simulink model "quadcopter_control_2018a"  (R2018a)
settings: Solver=VariableStepAuto  StartTime=0.0  StopTime=5.0  RelTol=1e-3
undefined symbols (not defined in the file or in its folder): armLength, b, dragFactor, iX, iY, iZ, J, Ke, Kt, mass, phi0, phiDot0, psi0, psiDot0, Ra, theta0, thetaDot0, thrustFactor, x0, xDot0, y0, yDot0, z0, zDot0
libraries: simulink x8
settings Model: Creator=Ramprasad  LastModifiedBy=BALA BASKAR
settings DebuggingCC: LibraryContextMissingDiagnostic=warning
settings SFSimCC: SimUseLocalCustomCode=on
settings RTWCC: RTWUseLocalCustomCode=on

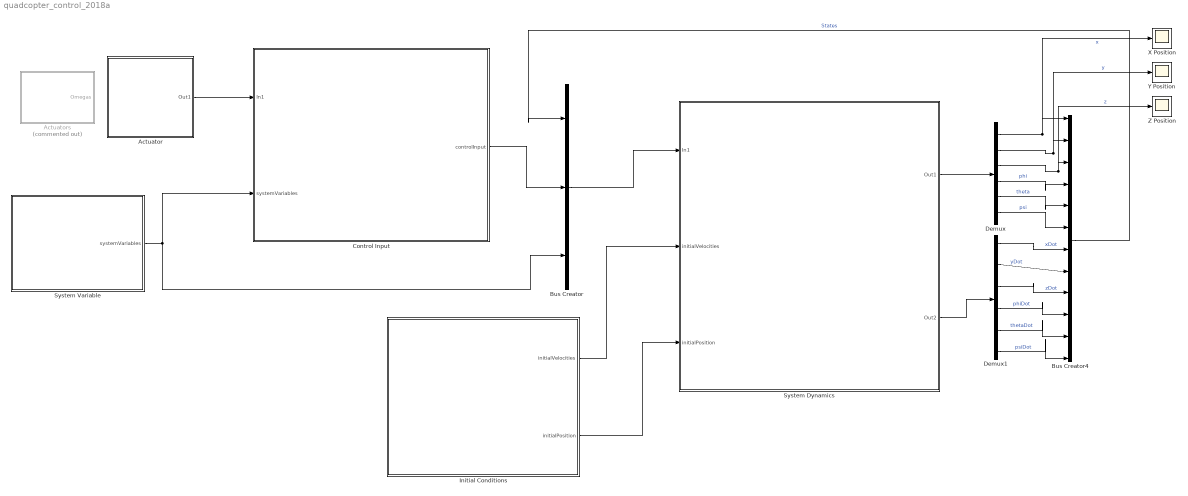
== system quadcopter_control_2018a ==
  Actuator : Subsystem
  Actuators : Subsystem  Commented=on
  Bus Creator : BusCreator  Inputs=3
  Bus Creator4 : BusCreator  Inputs=12
  Control Input : Subsystem
  Demux : Demux  Outputs=6
  Demux1 : Demux  Outputs=6
  Initial Conditions : Subsystem
  System Dynamics : Subsystem
  System Variable : Subsystem
  X Position : Scope
  Y Position : Scope
  Z Position : Scope
  wires:
  Bus Creator4/1 -> Bus Creator/1  "States"
  Demux/1 -> X Position/1, Bus Creator4/1  "x"
  Demux/2 -> Y Position/1, Bus Creator4/2  "y"
  Demux/3 -> Z Position/1, Bus Creator4/3  "z"
  Demux/4 -> Bus Creator4/4  "phi"
  Demux/5 -> Bus Creator4/5  "theta"
  Demux/6 -> Bus Creator4/6  "psi"
  Demux1/1 -> Bus Creator4/7  "xDot"
  Demux1/2 -> Bus Creator4/8  "yDot"
  Demux1/3 -> Bus Creator4/9  "zDot"
  Demux1/4 -> Bus Creator4/10  "phiDot"
  Demux1/5 -> Bus Creator4/11  "thetaDot"
  Demux1/6 -> Bus Creator4/12  "psiDot"
  Control Input/1(controlInput) -> Bus Creator/2
  Actuator/1(Out1) -> Control Input/1(In1)
  System Variable/1(systemVariables) -> Bus Creator/3, Control Input/2(systemVariables)
  Bus Creator/1 -> System Dynamics/1(In1)
  System Dynamics/1(Out1) -> Demux/1
  System Dynamics/2(Out2) -> Demux1/1
  Initial Conditions/1(initialVelocities) -> System Dynamics/2(initialVelocities)
  Initial Conditions/2(initialPosition) -> System Dynamics/3(initialPosition)

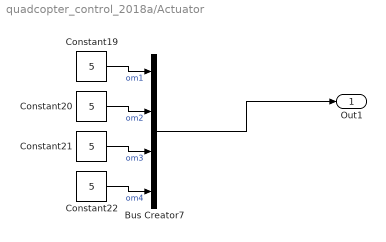
== system quadcopter_control_2018a/Actuator ==
  Bus Creator7 : BusCreator  Inputs=4
  Constant{19..22} (4 alike) : Constant  Value=5
  Out1 : Outport
  wires:
  Constant20/1 -> Bus Creator7/2  "om2"
  Bus Creator7/1 -> Out1/1
  Constant22/1 -> Bus Creator7/4  "om4"
  Constant21/1 -> Bus Creator7/3  "om3"
  Constant19/1 -> Bus Creator7/1  "om1"

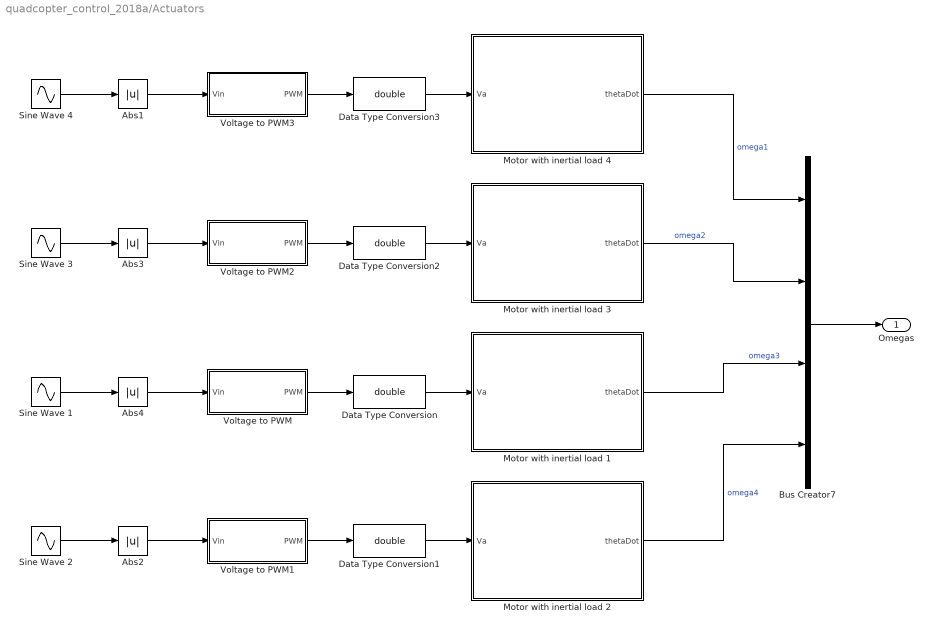
== system quadcopter_control_2018a/Actuators ==
  Abs{1..4} (4 alike) : Abs
  Bus Creator7 : BusCreator  Inputs=4
  Data Type Conversion{,1..3} (4 alike) : DataTypeConversion  OutDataTypeStr=double
  Motor with inertial load 1 : Subsystem
  Motor with inertial load 2 : Subsystem
  Motor with inertial load 3 : Subsystem
  Motor with inertial load 4 : Subsystem
  Sine Wave {1..4} (4 alike) : Sin  Amplitude=500  Frequency=50  SampleTime=0
  Voltage to PWM : Subsystem
  Voltage to PWM1 : Subsystem
  Voltage to PWM2 : Subsystem
  Voltage to PWM3 : Subsystem
  Omegas : Outport
  wires:
  Bus Creator7/1 -> Omegas/1
  Motor with inertial load 4/1(thetaDot) -> Bus Creator7/1  "omega1"
  Voltage to PWM2/1(PWM) -> Data Type Conversion2/1
  Sine Wave 1/1 -> Abs4/1
  Motor with inertial load 1/1(thetaDot) -> Bus Creator7/3  "omega3"
  Data Type Conversion3/1 -> Motor with inertial load 4/1(Va)
  Voltage to PWM/1(PWM) -> Data Type Conversion/1
  Sine Wave 3/1 -> Abs3/1
  Motor with inertial load 2/1(thetaDot) -> Bus Creator7/4  "omega4"
  Sine Wave 2/1 -> Abs2/1
  Voltage to PWM1/1(PWM) -> Data Type Conversion1/1
  Data Type Conversion2/1 -> Motor with inertial load 3/1(Va)
  Motor with inertial load 3/1(thetaDot) -> Bus Creator7/2  "omega2"
  Sine Wave 4/1 -> Abs1/1
  Data Type Conversion/1 -> Motor with inertial load 1/1(Va)
  Data Type Conversion1/1 -> Motor with inertial load 2/1(Va)
  Voltage to PWM3/1(PWM) -> Data Type Conversion3/1
  Abs1/1 -> Voltage to PWM3/1(Vin)
  Abs2/1 -> Voltage to PWM1/1(Vin)
  Abs3/1 -> Voltage to PWM2/1(Vin)
  Abs4/1 -> Voltage to PWM/1(Vin)

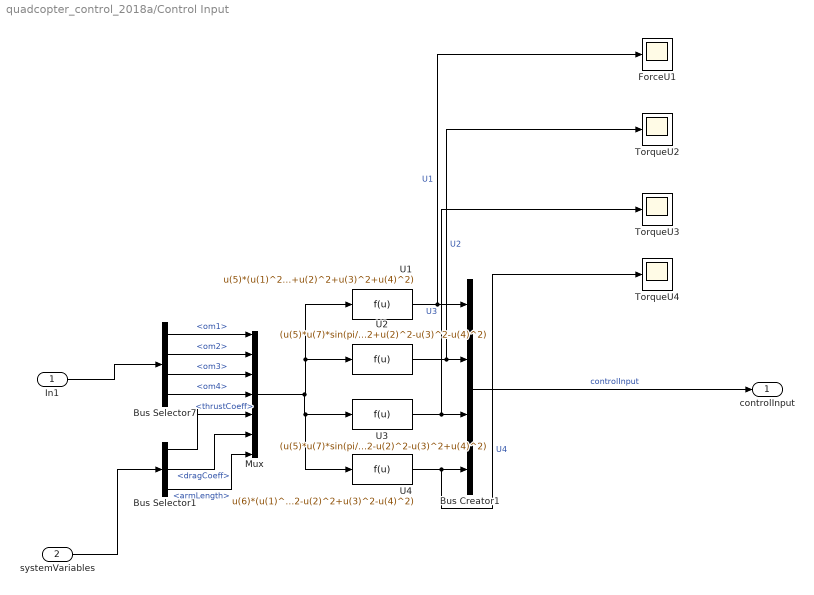
== system quadcopter_control_2018a/Control Input ==
  In1 : Inport
  systemVariables : Inport  Port=2
  Bus Creator1 : BusCreator  Inputs=4
  Bus Selector1 : BusSelector  OutputSignals=thrustCoeff,dragCoeff,armLength
  Bus Selector7 : BusSelector  OutputSignals=om1,om2,om3,om4
  ForceU1 : Scope
  Mux : Mux  Inputs=7
  TorqueU2 : Scope
  TorqueU3 : Scope
  TorqueU4 : Scope
  U1 : Fcn  Expr=u(5)*(u(1)^2+u(2)^2+u(3)^2+u(4)^2)
  U2 : Fcn  Expr=(u(5)*u(7)*sin(pi/4))*(u(1)^2+u(2)^2-u(3)^2-u(4)^2)
  U3 : Fcn  Expr=(u(5)*u(7)*sin(pi/4))*(u(1)^2-u(2)^2-u(3)^2+u(4)^2)
  U4 : Fcn  Expr=u(6)*(u(1)^2-u(2)^2+u(3)^2-u(4)^2)
  controlInput : Outport
  wires:
  systemVariables/1 -> Bus Selector1/1
  Bus Selector7/2 -> Mux/2  "<om2>"
  Bus Selector7/4 -> Mux/4  "<om4>"
  Bus Selector7/1 -> Mux/1  "<om1>"
  U2/1 -> TorqueU2/1, Bus Creator1/2  "U2"
  Bus Selector1/2 -> Mux/6  "<dragCoeff>"
  Bus Creator1/1 -> controlInput/1  "controlInput"
  Bus Selector1/1 -> Mux/5  "<thrustCoeff>"
  U3/1 -> TorqueU3/1, Bus Creator1/3  "U3"
  Bus Selector1/3 -> Mux/7  "<armLength>"
  U4/1 -> TorqueU4/1, Bus Creator1/4  "U4"
  U1/1 -> ForceU1/1, Bus Creator1/1  "U1"
  Mux/1 -> U4/1, U3/1, U2/1, U1/1
  In1/1 -> Bus Selector7/1
  Bus Selector7/3 -> Mux/3  "<om3>"

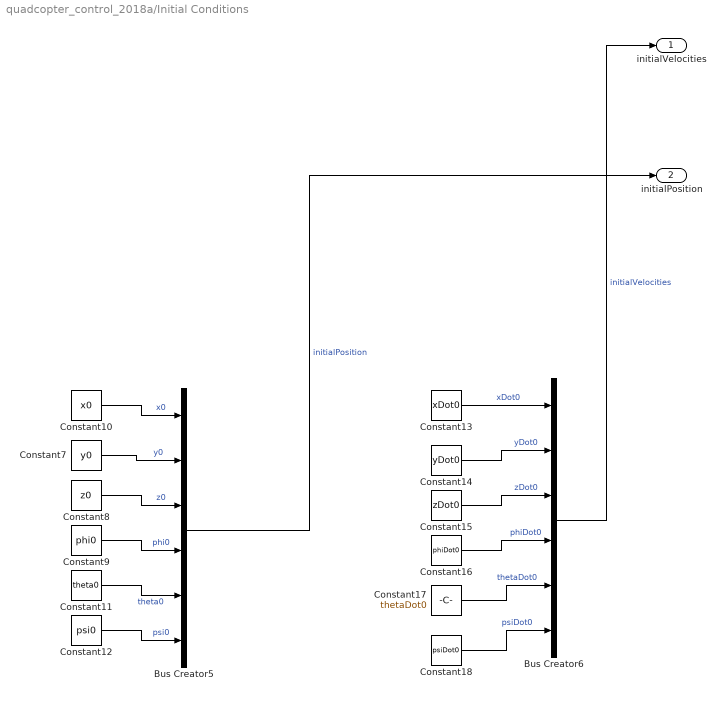
== system quadcopter_control_2018a/Initial Conditions ==
  Bus Creator5 : BusCreator  Inputs=6
  Bus Creator6 : BusCreator  Inputs=6
  Constant10 : Constant  Value=x0
  Constant11 : Constant  Value=theta0
  Constant12 : Constant  Value=psi0
  Constant13 : Constant  Value=xDot0
  Constant14 : Constant  Value=yDot0
  Constant15 : Constant  Value=zDot0
  Constant16 : Constant  Value=phiDot0
  Constant17 : Constant  Value=thetaDot0
  Constant18 : Constant  Value=psiDot0
  Constant7 : Constant  Value=y0
  Constant8 : Constant  Value=z0
  Constant9 : Constant  Value=phi0
  initialVelocities : Outport
  initialPosition : Outport  Port=2
  wires:
  Bus Creator5/1 -> initialPosition/1  "initialPosition"
  Constant7/1 -> Bus Creator5/2  "y0"
  Bus Creator6/1 -> initialVelocities/1  "initialVelocities"
  Constant10/1 -> Bus Creator5/1  "x0"
  Constant15/1 -> Bus Creator6/3  "zDot0"
  Constant12/1 -> Bus Creator5/6  "psi0"
  Constant16/1 -> Bus Creator6/4  "phiDot0"
  Constant8/1 -> Bus Creator5/3  "z0"
  Constant11/1 -> Bus Creator5/5  "theta0"
  Constant13/1 -> Bus Creator6/1  "xDot0"
  Constant18/1 -> Bus Creator6/6  "psiDot0"
  Constant17/1 -> Bus Creator6/5  "thetaDot0"
  Constant14/1 -> Bus Creator6/2  "yDot0"
  Constant9/1 -> Bus Creator5/4  "phi0"

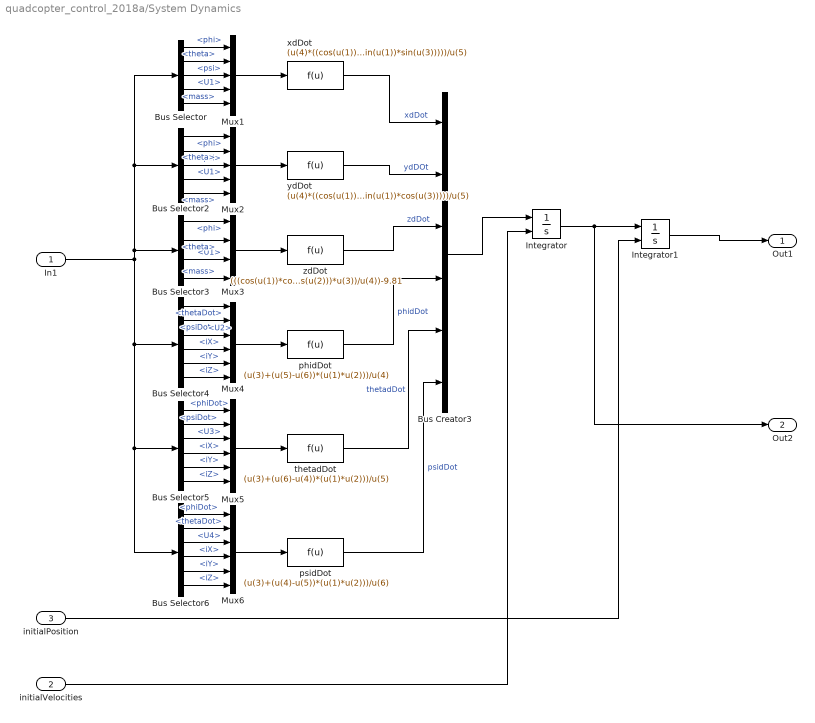
== system quadcopter_control_2018a/System Dynamics ==
  In1 : Inport
  initialVelocities : Inport  Port=2
  initialPosition : Inport  Port=3
  Bus Creator3 : BusCreator  Inputs=6
  Bus Selector : BusSelector  OutputSignals=States.phi,States.theta,States.psi,controlInput.U1,systemVariables.mass
  Bus Selector2 : BusSelector  OutputSignals=States.phi,States.theta,States.psi,controlInput.U1,systemVariables.mass
  Bus Selector3 : BusSelector  OutputSignals=States.phi,States.theta,controlInput.U1,systemVariables.mass
  Bus Selector4 : BusSelector  OutputSignals=States.thetaDot,States.psiDot,controlInput.U2,systemVariables.iX,systemVariables.iY,systemVariables.iZ
  Bus Selector5 : BusSelector  OutputSignals=States.phiDot,States.psiDot,controlInput.U3,systemVariables.iX,systemVariables.iY,systemVariables.iZ
  Bus Selector6 : BusSelector  OutputSignals=States.phiDot,States.thetaDot,controlInput.U4,systemVariables.iX,systemVariables.iY,systemVariables.iZ
  Integrator : Integrator  InitialConditionSource=external
  Integrator1 : Integrator  InitialConditionSource=external
  Mux1 : Mux  Inputs=5
  Mux2 : Mux  Inputs=5
  Mux3 : Mux
  Mux4 : Mux  Inputs=6
  Mux5 : Mux  Inputs=6
  Mux6 : Mux  Inputs=6
  phidDot : Fcn  Expr=(u(3)+(u(5)-u(6))*(u(1)*u(2)))/u(4)
  psidDot : Fcn  Expr=(u(3)+(u(4)-u(5))*(u(1)*u(2)))/u(6)
  thetadDot : Fcn  Expr=(u(3)+(u(6)-u(4))*(u(1)*u(2)))/u(5)
  xdDot : Fcn  Expr=(u(4)*((cos(u(1))*sin(u(2))*cos(u(3)))+(sin(u(1))*sin(u(3)))))/u(5)
  ydDot : Fcn  Expr=(u(4)*((cos(u(1))*sin(u(2))*sin(u(3)))-(sin(u(1))*cos(u(3)))))/u(5)
  zdDot : Fcn  Expr=(((cos(u(1))*cos(u(2)))*u(3))/u(4))-9.81
  Out1 : Outport
  Out2 : Outport  Port=2
  wires:
  Mux1/1 -> xdDot/1
  Bus Selector3/4 -> Mux3/4  "<mass>"
  Bus Selector/2 -> Mux1/2  "<theta>"
  Bus Selector5/5 -> Mux5/5  "<iY>"
  ydDot/1 -> Bus Creator3/2  "ydDOt"
  Bus Selector/5 -> Mux1/5  "<mass>"
  Integrator1/1 -> Out1/1
  psidDot/1 -> Bus Creator3/6  "psidDot"
  Integrator/1 -> Out2/1, Integrator1/1
  Mux3/1 -> zdDot/1
  Bus Selector4/1 -> Mux4/1  "<thetaDot>"
  Bus Selector4/4 -> Mux4/4  "<iX>"
  Bus Selector6/5 -> Mux6/5  "<iY>"
  Bus Selector4/2 -> Mux4/2  "<psiDot>"
  Bus Selector5/1 -> Mux5/1  "<phiDot>"
  zdDot/1 -> Bus Creator3/3  "zdDot"
  Bus Selector6/1 -> Mux6/1  "<phiDot>"
  Bus Selector6/3 -> Mux6/3  "<U4>"
  Mux2/1 -> ydDot/1
  Bus Selector3/3 -> Mux3/3  "<U1>"
  Bus Selector6/6 -> Mux6/6  "<iZ>"
  Bus Creator3/1 -> Integrator/1
  Bus Selector2/5 -> Mux2/5  "<mass>"
  Bus Selector4/6 -> Mux4/6  "<iZ>"
  Mux4/1 -> phidDot/1
  Bus Selector/1 -> Mux1/1  "<phi>"
  Bus Selector/4 -> Mux1/4  "<U1>"
  Bus Selector5/4 -> Mux5/4  "<iX>"
  Mux6/1 -> psidDot/1
  Bus Selector/3 -> Mux1/3  "<psi>"
  initialVelocities/1 -> Integrator/2
  Bus Selector3/1 -> Mux3/1  "<phi>"
  Bus Selector3/2 -> Mux3/2  "<theta>"
  Bus Selector5/3 -> Mux5/3  "<U3>"
  In1/1 -> Bus Selector/1, Bus Selector2/1, Bus Selector3/1, Bus Selector6/1, Bus Selector5/1, Bus Selector4/1
  Bus Selector2/3 -> Mux2/3  "<psi>"
  phidDot/1 -> Bus Creator3/4  "phidDot"
  Bus Selector6/2 -> Mux6/2  "<thetaDot>"
  Bus Selector5/6 -> Mux5/6  "<iZ>"
  Bus Selector6/4 -> Mux6/4  "<iX>"
  Mux5/1 -> thetadDot/1
  Bus Selector2/1 -> Mux2/1  "<phi>"
  Bus Selector5/2 -> Mux5/2  "<psiDot>"
  thetadDot/1 -> Bus Creator3/5  "thetadDot"
  Bus Selector4/3 -> Mux4/3  "<U2>"
  Bus Selector2/4 -> Mux2/4  "<U1>"
  Bus Selector4/5 -> Mux4/5  "<iY>"
  Bus Selector2/2 -> Mux2/2  "<theta>"
  xdDot/1 -> Bus Creator3/1  "xdDot"
  initialPosition/1 -> Integrator1/2

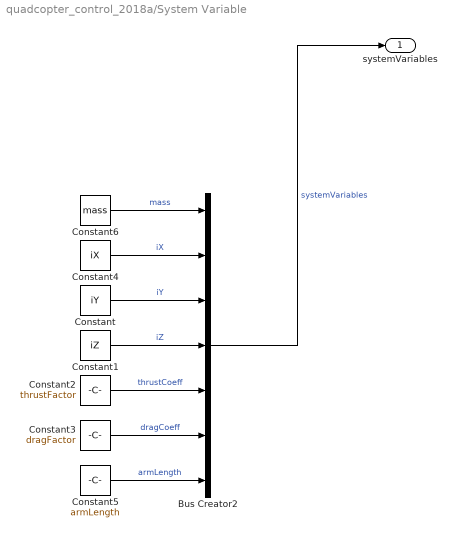
== system quadcopter_control_2018a/System Variable ==
  Bus Creator2 : BusCreator  Inputs=7
  Constant : Constant  Value=iY
  Constant1 : Constant  Value=iZ
  Constant2 : Constant  Value=thrustFactor
  Constant3 : Constant  Value=dragFactor
  Constant4 : Constant  Value=iX
  Constant5 : Constant  Value=armLength
  Constant6 : Constant  Value=mass
  systemVariables : Outport
  wires:
  Bus Creator2/1 -> systemVariables/1  "systemVariables"
  Constant5/1 -> Bus Creator2/7  "armLength"
  Constant4/1 -> Bus Creator2/2  "iX"
  Constant3/1 -> Bus Creator2/6  "dragCoeff"
  Constant1/1 -> Bus Creator2/4  "iZ"
  Constant/1 -> Bus Creator2/3  "iY"
  Constant2/1 -> Bus Creator2/5  "thrustCoeff"
  Constant6/1 -> Bus Creator2/1  "mass"

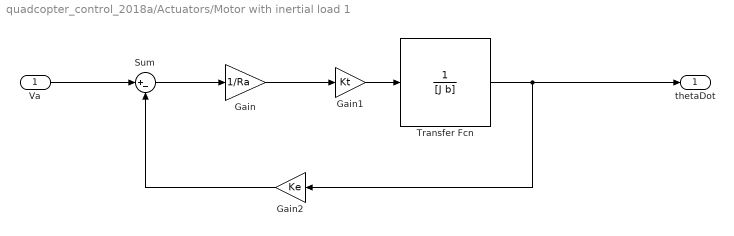
== system quadcopter_control_2018a/Actuators/Motor with inertial load 1 ==
  Va : Inport
  Gain : Gain  Gain=1/Ra
  Gain1 : Gain  Gain=Kt
  Gain2 : Gain  Gain=Ke
  Sum : Sum  Inputs=|+-
  Transfer Fcn : TransferFcn  Denominator=[J b]
  thetaDot : Outport
  wires:
  Va/1 -> Sum/1
  Transfer Fcn/1 -> thetaDot/1, Gain2/1
  Gain1/1 -> Transfer Fcn/1
  Gain2/1 -> Sum/2
  Gain/1 -> Gain1/1
  Sum/1 -> Gain/1

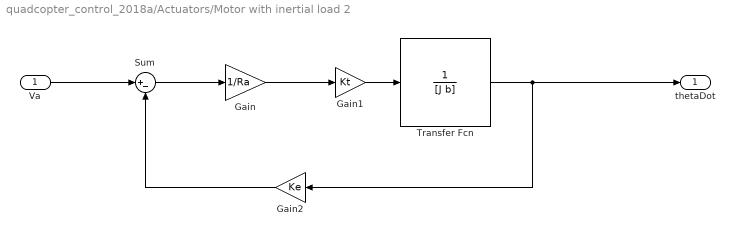
== system quadcopter_control_2018a/Actuators/Motor with inertial load 2 ==
  Va : Inport
  Gain : Gain  Gain=1/Ra
  Gain1 : Gain  Gain=Kt
  Gain2 : Gain  Gain=Ke
  Sum : Sum  Inputs=|+-
  Transfer Fcn : TransferFcn  Denominator=[J b]
  thetaDot : Outport
  wires:
  Va/1 -> Sum/1
  Transfer Fcn/1 -> thetaDot/1, Gain2/1
  Gain1/1 -> Transfer Fcn/1
  Gain2/1 -> Sum/2
  Gain/1 -> Gain1/1
  Sum/1 -> Gain/1

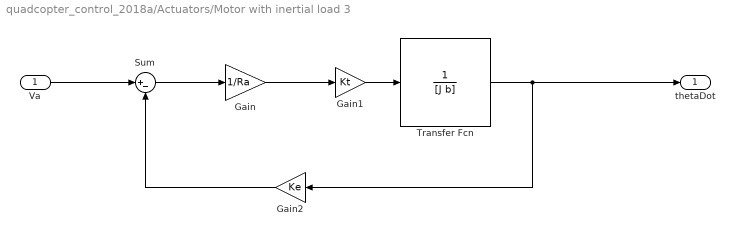
== system quadcopter_control_2018a/Actuators/Motor with inertial load 3 ==
  Va : Inport
  Gain : Gain  Gain=1/Ra
  Gain1 : Gain  Gain=Kt
  Gain2 : Gain  Gain=Ke
  Sum : Sum  Inputs=|+-
  Transfer Fcn : TransferFcn  Denominator=[J b]
  thetaDot : Outport
  wires:
  Va/1 -> Sum/1
  Transfer Fcn/1 -> thetaDot/1, Gain2/1
  Gain1/1 -> Transfer Fcn/1
  Gain2/1 -> Sum/2
  Gain/1 -> Gain1/1
  Sum/1 -> Gain/1

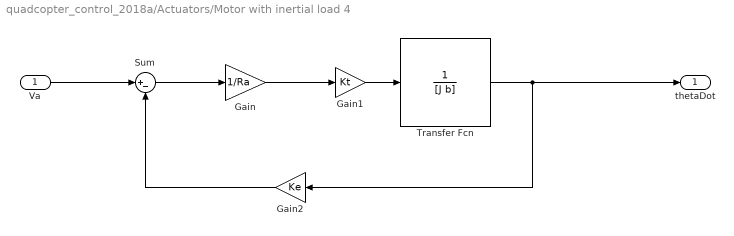
== system quadcopter_control_2018a/Actuators/Motor with inertial load 4 ==
  Va : Inport
  Gain : Gain  Gain=1/Ra
  Gain1 : Gain  Gain=Kt
  Gain2 : Gain  Gain=Ke
  Sum : Sum  Inputs=|+-
  Transfer Fcn : TransferFcn  Denominator=[J b]
  thetaDot : Outport
  wires:
  Va/1 -> Sum/1
  Transfer Fcn/1 -> thetaDot/1, Gain2/1
  Gain1/1 -> Transfer Fcn/1
  Gain2/1 -> Sum/2
  Gain/1 -> Gain1/1
  Sum/1 -> Gain/1

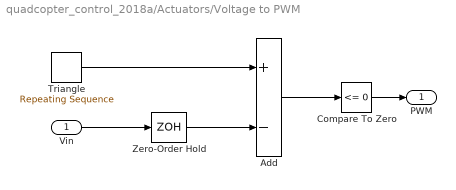
== system quadcopter_control_2018a/Actuators/Voltage to PWM ==
  Vin : Inport
  Add : Sum  Inputs=+-  SampleTime=1/10000
  Compare To Zero : simulink/Logic and Bit Operations/Compare To Zero  relop=<=  OutDataTypeStr=uint8
  Triangle : simulink/Sources/Repeating Sequence  rep_seq_t=[0 1/100/4 3/100/4 1/100]*25  rep_seq_y=[0.5 0 1 0.5]
  Zero-Order Hold : ZeroOrderHold  SampleTime=1/10000
  PWM : Outport
  wires:
  Triangle/1 -> Add/1
  Vin/1 -> Zero-Order Hold/1
  Add/1 -> Compare To Zero/1
  Compare To Zero/1 -> PWM/1
  Zero-Order Hold/1 -> Add/2

== system quadcopter_control_2018a/Actuators/Voltage to PWM1 ==
  Vin : Inport
  Add : Sum  Inputs=+-  SampleTime=1/10000
  Compare To Zero : simulink/Logic and Bit Operations/Compare To Zero  relop=<=  OutDataTypeStr=uint8
  Triangle : simulink/Sources/Repeating Sequence  rep_seq_t=[0 1/100/4 3/100/4 1/100]*25  rep_seq_y=[0.5 0 1 0.5]
  Zero-Order Hold : ZeroOrderHold  SampleTime=1/10000
  PWM : Outport
  wires:
  Triangle/1 -> Add/1
  Vin/1 -> Zero-Order Hold/1
  Add/1 -> Compare To Zero/1
  Compare To Zero/1 -> PWM/1
  Zero-Order Hold/1 -> Add/2

== system quadcopter_control_2018a/Actuators/Voltage to PWM2 ==
  Vin : Inport
  Add : Sum  Inputs=+-  SampleTime=1/10000
  Compare To Zero : simulink/Logic and Bit Operations/Compare To Zero  relop=<=  OutDataTypeStr=uint8
  Triangle : simulink/Sources/Repeating Sequence  rep_seq_t=[0 1/100/4 3/100/4 1/100]*25  rep_seq_y=[0.5 0 1 0.5]
  Zero-Order Hold : ZeroOrderHold  SampleTime=1/10000
  PWM : Outport
  wires:
  Triangle/1 -> Add/1
  Vin/1 -> Zero-Order Hold/1
  Add/1 -> Compare To Zero/1
  Compare To Zero/1 -> PWM/1
  Zero-Order Hold/1 -> Add/2

== system quadcopter_control_2018a/Actuators/Voltage to PWM3 ==
  Vin : Inport
  Add : Sum  Inputs=+-  SampleTime=1/10000
  Compare To Zero : simulink/Logic and Bit Operations/Compare To Zero  relop=<=  OutDataTypeStr=uint8
  Triangle : simulink/Sources/Repeating Sequence  rep_seq_t=[0 1/100/4 3/100/4 1/100]*5  rep_seq_y=[0.5 0 1 0.5]
  Zero-Order Hold : ZeroOrderHold  SampleTime=1/10000
  PWM : Outport
  wires:
  Triangle/1 -> Add/1
  Vin/1 -> Zero-Order Hold/1
  Add/1 -> Compare To Zero/1
  Compare To Zero/1 -> PWM/1
  Zero-Order Hold/1 -> Add/2
